simulink model "newww"  (R2019a)
settings: Solver=VariableStepAuto  StartTime=0.0  StopTime=770  RelTol=1e-3
undefined symbols (not defined in the file or in its folder): Ion, Lithium
libraries: powerlib x11, electricdrivelib x3
settings Model: SimulationMode=accelerator  Creator=rachad  LastModifiedBy=رشاد
settings SolverCC: ZeroCrossAlgorithm=Adaptive
settings DebuggingCC: IgnoredZcDiagnostic=none

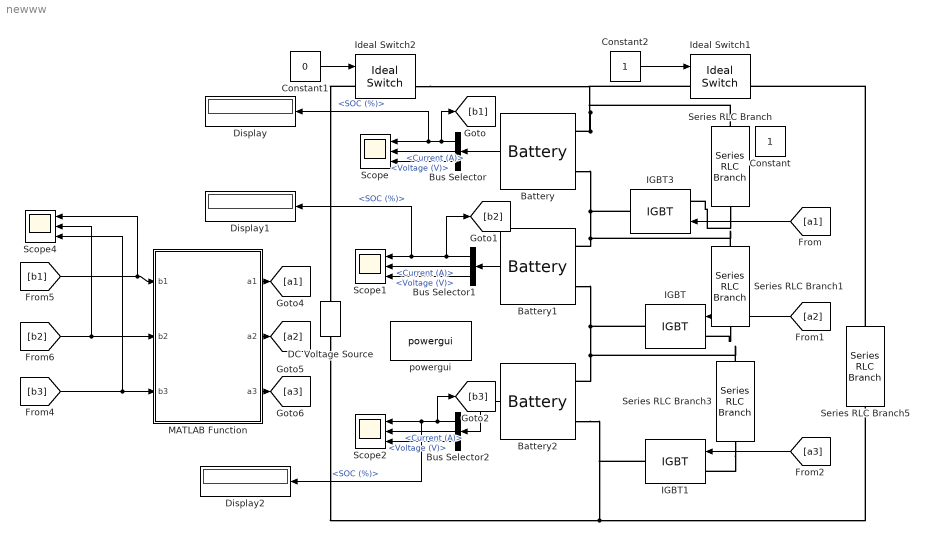
== system newww ==
  Battery : electricdrivelib/Extra Sources/Battery  BatType=Lithium-Ion  ShowTempParam=off  ThermalPreset=no  ShowAgeParam=off  NomV=3.6  NomQ=2.6  SOC=100  Batt_Tr=10  PresetModel=on  MaxQ=2.6  MinV=2.7  FullV=4.1904  Dis_rate=1.1304  R=0.013846  Normal_OP=2.3513  expZone="[3.8894     0.12774]"  current=[6.5 13 32.5]  Units=Time  Tci=20  NomT=20  T2=-30  MaxQ2=4.8  FullV2=7.1  Normal_OP2=5.655  expZone2="[6.58           1]"  Rca=0.6  ti=2000  Dp=0  Neq0=0  Tsim=1e6  Ta1=25  Qeol=5.4*0.9  Reol=0.013333*1.2  Char_age=[2.3478, 3]  Dis_age=[2.3478, 10]  N1=1500  N2=10500  N3=1000  N4=1400  Ta2=45  N5=950
      settings: SourceProductName=Simscape Electrical
  Battery1 : electricdrivelib/Extra Sources/Battery  BatType=Lithium-Ion  ShowTempParam=off  ThermalPreset=no  ShowAgeParam=off  NomV=3.6  NomQ=2.6  SOC=75  Batt_Tr=10  PresetModel=on  MaxQ=2.6  MinV=2.7  FullV=4.1904  Dis_rate=1.1304  R=0.013846  Normal_OP=2.3513  expZone="[3.8894     0.12774]"  current=[6.5 13 32.5]  Units=Time  Tci=20  NomT=20  T2=-30  MaxQ2=4.8  FullV2=7.1  Normal_OP2=5.655  expZone2="[6.58           1]"  Rca=0.6  ti=2000  Dp=0  Neq0=0  Tsim=1e6  Ta1=25  Qeol=5.4*0.9  Reol=0.013333*1.2  Char_age=[2.3478, 3]  Dis_age=[2.3478, 10]  N1=1500  N2=10500  N3=1000  N4=1400  Ta2=45  N5=950
      settings: SourceProductName=Simscape Electrical
  Battery2 : electricdrivelib/Extra Sources/Battery  BatType=Lithium-Ion  ShowTempParam=off  ThermalPreset=no  ShowAgeParam=off  NomV=3.6  NomQ=2.6  SOC=97  Batt_Tr=10  PresetModel=on  MaxQ=2.6  MinV=2.7  FullV=4.1904  Dis_rate=1.1304  R=0.013846  Normal_OP=2.3513  expZone="[3.8894     0.12774]"  current=[6.5 13 32.5]  Units=Time  Tci=20  NomT=20  T2=-30  MaxQ2=4.8  FullV2=7.1  Normal_OP2=5.655  expZone2="[6.58           1]"  Rca=0.6  ti=2000  Dp=0  Neq0=0  Tsim=1e6  Ta1=25  Qeol=5.4*0.9  Reol=0.013333*1.2  Char_age=[2.3478, 3]  Dis_age=[2.3478, 10]  N1=1500  N2=10500  N3=1000  N4=1400  Ta2=45  N5=950
      settings: SourceProductName=Simscape Electrical
  Bus Selector : BusSelector  OutputSignals=SOC (%),Current (A),Voltage (V)
  Bus Selector1 : BusSelector  OutputSignals=SOC (%),Current (A),Voltage (V)
  Bus Selector2 : BusSelector  OutputSignals=SOC (%),Current (A),Voltage (V)
  Constant : Constant
  Constant1 : Constant  Value=0
  Constant2 : Constant
  DC Voltage Source : powerlib/Electrical Sources/DC Voltage Source  Amplitude=14  Measurements=None
      settings: SourceProductName=Simscape Electrical
  Display : Display
  Display1 : Display
  Display2 : Display
  IGBT : powerlib/Power Electronics/IGBT  Ron=0  Lon=0  Vf=1  Tf=1e-6  Tt=2e-6  IC=0  Rs=1e-05  Cs=0  Measurements=off
      settings: SourceProductName=Simscape Electrical
  IGBT1 : powerlib/Power Electronics/IGBT  Ron=0  Lon=0  Vf=1  Tf=1e-6  Tt=2e-6  IC=0  Rs=1e-05  Cs=0  Measurements=off
      settings: SourceProductName=Simscape Electrical
  IGBT3 : powerlib/Power Electronics/IGBT  Ron=0.001  Lon=0  Vf=1  Tf=1e-6  Tt=2e-6  IC=0  Rs=1e-05  Cs=0  Measurements=off
      settings: SourceProductName=Simscape Electrical
  Ideal Switch1 : powerlib/Power Electronics/Ideal Switch  Ron=0.001  Lon=0  IC=0  Rs=1e5  Cs=inf  Measurements=on
      settings: SourceProductName=Simscape Electrical
  Ideal Switch2 : powerlib/Power Electronics/Ideal Switch  Ron=0.001  Lon=0  IC=0  Rs=1e5  Cs=inf  Measurements=on
      settings: SourceProductName=Simscape Electrical
  MATLAB Function : MATLAB Function  TreatAsAtomicUnit=on
  Scope{,1..2,4} (4 alike) : Scope  NumInputPorts=3
  Series RLC Branch{,1,3,5} (4 alike) : powerlib/Elements/Series RLC Branch  LConnTagsString=__new0  RConnTagsString=__new0  BranchType=R  Resistance=1  Inductance=1e-3  SetiL0=off  InitialCurrent=0  Capacitance=1e-6  Setx0=off  InitialVoltage=0  Measurements=None
      settings: SourceProductName=Simscape Electrical
  powergui : powerlib/powergui  Priority=1  SimulationMode=Continuous  SampleTime=50e-6  frequency=60  Iterations=50  frequencyindice=0  Pbase=100e6  ErrMax=1e-4  UnitsV=kV  UnitsW=MW  buscounter=0  FunctionMessages=off  echomessages=off  EnableUseOfTLC=off  CurrentSourceSwitches=off  DisableSnubberDevices=off  DisableRonSwitches=off  DisableVfSwitches=off  DisplayEquations=off  AutomaticDiscreteSolvers=off  SolverType=Tustin/Backward Euler (TBE)  Interpol=off  ExternalGateDelay=off  methode=off  Ts=100  x0status=blocks  SPID=on  SwTol=0  HookPort=off  NonlinearTolerance=0  nMaxIteration=15  ContinueOnMaxIteration=off  RestoreLinks=warning  ResistiveCurrentMeasurement=off  Frange=[0:2:500]  Ylog=off  Xlog=on  ShowGrid=off  save=off  variable=ZData  structure=0  ZoomFFT=off  StartTime=0.0  cycles=1  DisplayStyle=1  fundamental=60  FreqAxis=off  MaxFrequency=1000  frequencyindicesteady=1  RmsSteady=1  display=off
      settings: SourceProductName=Simscape Electrical
  wires:
  Battery/1 -> Bus Selector/1
  Battery1/1 -> Bus Selector1/1
  Battery2/1 -> Bus Selector2/1
  Bus Selector/1 -> [b1], Display/1, Scope/1  "<SOC (%)>"
  Bus Selector/3 -> Scope/3  "<Voltage (V)>"
  Constant1/1 -> Ideal Switch2/1
  Constant2/1 -> Ideal Switch1/1
  Bus Selector/2 -> Scope/2  "<Current (A)>"
  Bus Selector1/3 -> Scope1/3  "<Voltage (V)>"
  Bus Selector1/2 -> Scope1/2  "<Current (A)>"
  Bus Selector2/1 -> [b3], Display2/1, Scope2/1  "<SOC (%)>"
  Bus Selector2/2 -> Scope2/2  "<Current (A)>"
  Bus Selector2/3 -> Scope2/3  "<Voltage (V)>"
  Bus Selector1/1 -> [b2], Display1/1, Scope1/1  "<SOC (%)>"
  MATLAB Function/3(a3) -> [a3]
  MATLAB Function/1(a1) -> [a1]
  MATLAB Function/2(a2) -> [a2]
  [b1] -> Scope4/1, MATLAB Function/1(b1)
  [b3] -> MATLAB Function/3(b3), Scope4/3
  [b2] -> MATLAB Function/2(b2), Scope4/2
  [a1] -> IGBT3/1
  [a2] -> IGBT/1
  [a3] -> IGBT1/1
  connections:
  Battery/LConn2 -- IGBT3/RConn1 -- Battery1/LConn1 -- Series RLC Branch1/LConn1
  Battery1/LConn2 -- IGBT/RConn1 -- Battery2/LConn1 -- Series RLC Branch3/LConn1
  Battery/LConn1 -- Ideal Switch1/LConn1 -- Ideal Switch2/RConn1 -- Series RLC Branch/LConn1
  DC Voltage Source/LConn1 -- Battery2/LConn2 -- IGBT1/RConn1 -- Series RLC Branch5/RConn1
  Series RLC Branch1/RConn1 -- IGBT/LConn1
  Series RLC Branch3/RConn1 -- IGBT1/LConn1
  Series RLC Branch5/LConn1 -- Ideal Switch1/RConn1
  Series RLC Branch/RConn1 -- IGBT3/LConn1
  Ideal Switch2/LConn1 -- DC Voltage Source/RConn1

== matlab function newww/MATLAB Function ==
  data: a1 output; a2 output; b1 input; b2 input; b3 input; a3 output
function [a1, a2, a3] = fcn(b1, b2, b3)

b1 = b1*1000;
b2 = b2*1000;
b3 = b3*1000;


b1 = int32(b1);
b2 = int32(b2);
b3 = int32(b3);
%t=max([b1 b2 b3]);

if max([b1 b2 b3])== b1
    a1=1;
    else
    a1=0;
end
if max([b1 b2 b3])== b2
    a2=1;
    else
    a2=0;
end
if max([b1 b2 b3])== b3
    a3=1;
    else
    a3=0;
end
if b1==b2 && b2==b3
    a1=0;
    a2=0;
    a3=0;

    
%if((b1>b2) || (b1>b3) )
%    a1=1;
%else
%    a1=0;
%end

%if (b2>b1 || b2>b3 )
  %  a2=1;
%else
  %  a2=0;
%end

%if (b3>b1 || b3>b2 )
  %  a3=1;
%else
 %   a3=0;
%end


end

end
